simulink model "my_stanley"  (R2020a)
settings: Solver=FixedStepAuto  StartTime=0.0  StopTime=20  FixedStep=.01  RelTol=1e-3
libraries: simulink x2
settings Model: Creator=Jamie  LastModifiedBy=Jamie
settings SolverCC: AlgebraicLoopSolver=LineSearch

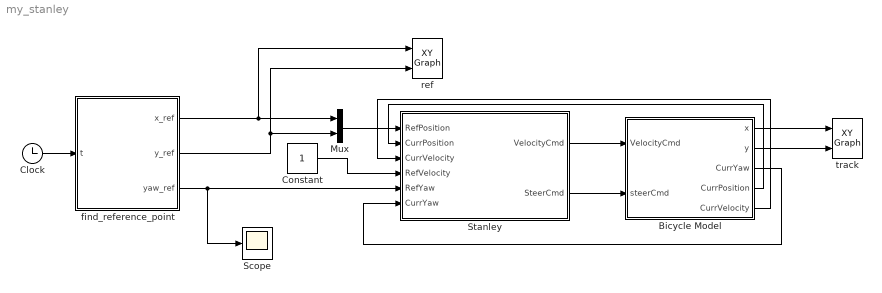
== system my_stanley ==
  Bicycle Model : Subsystem
  Clock : Clock
  Constant : Constant
  Mux : Mux  Inputs=2
  Scope : Scope
  Stanley : Subsystem
  find_reference_point : MATLAB Function  TreatAsAtomicUnit=on
  ref : simulink/Sinks/XY Graph  xmin=-4  xmax=4  ymin=-3  ymax=3  st=-1
  track : simulink/Sinks/XY Graph  xmin=-4  xmax=4  ymin=-3  ymax=3  st=-1
  wires:
  Mux/1 -> Stanley/1(RefPosition)
  Bicycle Model/4(CurrPosition) -> Stanley/2(CurrPosition)
  Stanley/2(SteerCmd) -> Bicycle Model/2(steerCmd)
  Bicycle Model/3(CurrYaw) -> Stanley/6(CurrYaw)
  Bicycle Model/1(x) -> track/1
  Bicycle Model/2(y) -> track/2
  Stanley/1(VelocityCmd) -> Bicycle Model/1(VelocityCmd)
  find_reference_point/1(x_ref) -> ref/1, Mux/1
  find_reference_point/2(y_ref) -> ref/2, Mux/2
  Clock/1 -> find_reference_point/1(t)
  find_reference_point/3(yaw_ref) -> Scope/1, Stanley/5(RefYaw)
  Bicycle Model/5(CurrVelocity) -> Stanley/3(CurrVelocity)
  Constant/1 -> Stanley/4(RefVelocity)

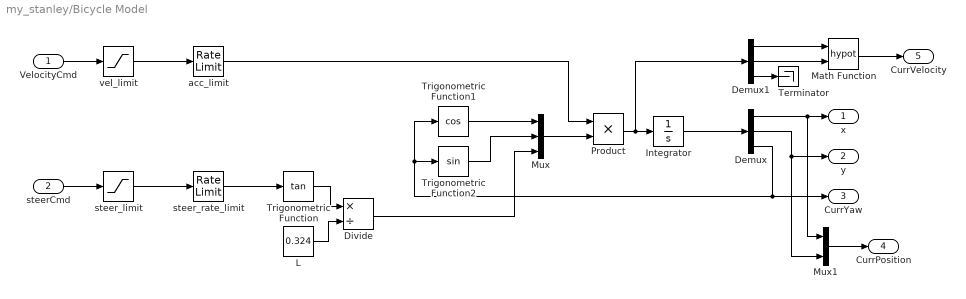
== system my_stanley/Bicycle Model ==
  VelocityCmd : Inport
  steerCmd : Inport  Port=2
  Demux : Demux  Outputs=3
  Demux1 : Demux  Outputs=3
  Divide : Product  Inputs=*/
  Integrator : Integrator  InitialCondition=[0, 0, pi/2]
  L : Constant  Value=0.324
  Math Function : Math  Operator=hypot  SaturateOnIntegerOverflow=on
  Mux : Mux  Inputs=3
  Mux1 : Mux  Inputs=2
  Product : Product
  Terminator : Terminator
  Trigonometric Function : Trigonometry  Operator=tan
  Trigonometric Function1 : Trigonometry  Operator=cos
  Trigonometric Function2 : Trigonometry
  acc_limit : RateLimiter  SampleTimeMode=inherited
  steer_limit : Saturate
  steer_rate_limit : RateLimiter  RisingSlewLimit=3  FallingSlewLimit=-3  SampleTimeMode=inherited
  vel_limit : Saturate  UpperLimit=3  LowerLimit=-3
  x : Outport
  y : Outport  Port=2
  CurrYaw : Outport  Port=3
  CurrPosition : Outport  Port=4
  CurrVelocity : Outport  Port=5
  wires:
  steerCmd/1 -> steer_limit/1
  VelocityCmd/1 -> vel_limit/1
  vel_limit/1 -> acc_limit/1
  steer_limit/1 -> steer_rate_limit/1
  steer_rate_limit/1 -> Trigonometric Function/1
  Trigonometric Function/1 -> Divide/1
  L/1 -> Divide/2
  acc_limit/1 -> Product/1
  Trigonometric Function1/1 -> Mux/1
  Trigonometric Function2/1 -> Mux/2
  Mux/1 -> Product/2
  Product/1 -> Demux1/1, Integrator/1
  Divide/1 -> Mux/3
  Integrator/1 -> Demux/1
  Demux/1 -> Mux1/1, x/1
  Demux/2 -> Mux1/2, y/1
  Demux/3 -> Trigonometric Function1/1, Trigonometric Function2/1, CurrYaw/1
  Mux1/1 -> CurrPosition/1
  Demux1/2 -> Math Function/2
  Demux1/1 -> Math Function/1
  Math Function/1 -> CurrVelocity/1
  Demux1/3 -> Terminator/1

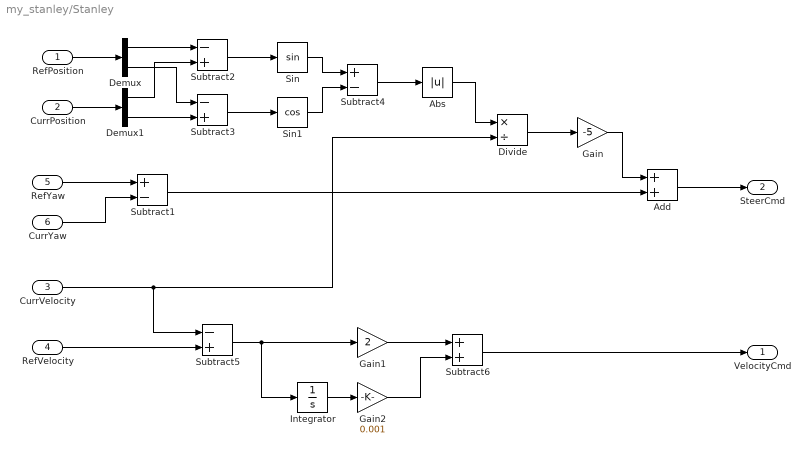
== system my_stanley/Stanley ==
  RefPosition : Inport
  CurrPosition : Inport  Port=2
  CurrVelocity : Inport  Port=3
  RefVelocity : Inport  Port=4
  RefYaw : Inport  Port=5
  CurrYaw : Inport  Port=6
  Abs : Abs
  Add : Sum
  Demux : Demux  Outputs=2
  Demux1 : Demux  Outputs=2
  Divide : Product  Inputs=*/
  Gain : Gain  Gain=-5
  Gain1 : Gain  Gain=2
  Gain2 : Gain  Gain=0.001
  Integrator : Integrator  InitialCondition=0.00001
  Sin : Trigonometry
  Sin1 : Trigonometry  Operator=cos
  Subtract1 : Sum  Inputs=+-
  Subtract2 : Sum  Inputs=-+
  Subtract3 : Sum  Inputs=-+
  Subtract4 : Sum  Inputs=+-
  Subtract5 : Sum  Inputs=-+
  Subtract6 : Sum
  VelocityCmd : Outport
  SteerCmd : Outport  Port=2
  wires:
  RefPosition/1 -> Demux/1
  RefYaw/1 -> Subtract1/1
  CurrYaw/1 -> Subtract1/2
  Add/1 -> SteerCmd/1
  Subtract1/1 -> Add/2
  CurrPosition/1 -> Demux1/1
  Demux1/1 -> Subtract2/2
  Demux/1 -> Subtract2/1
  Subtract2/1 -> Sin/1
  Demux1/2 -> Subtract3/2
  Demux/2 -> Subtract3/1
  Subtract3/1 -> Sin1/1
  Subtract4/1 -> Abs/1
  Sin/1 -> Subtract4/1
  Sin1/1 -> Subtract4/2
  Abs/1 -> Divide/1
  CurrVelocity/1 -> Subtract5/1, Divide/2
  Divide/1 -> Gain/1
  Gain/1 -> Add/1
  RefVelocity/1 -> Subtract5/2
  Subtract5/1 -> Integrator/1, Gain1/1
  Integrator/1 -> Gain2/1
  Subtract6/1 -> VelocityCmd/1
  Gain1/1 -> Subtract6/1
  Gain2/1 -> Subtract6/2

== matlab function my_stanley/find_reference_point ==
  data: t input; x_ref output; y_ref output; yaw_ref output
function [x_ref, y_ref, yaw_ref]= fcn(t)
pi = 3.14159;

v = 1;
R = 1.5;
T0 = pi*R/v;

if (t>4*T0)
    t = mod(t,(4*T0));
end
    
if ((t >= 0)&&(t <= 2*T0))
    x_ref = R + R*cos(pi - (v/R)*t);
    y_ref = R*sin(pi - (v/R)*t);
    yaw_ref = pi/2 - (v/R)*t;
elseif ((t >= 2*T0)&&(t <= 4*T0))
    x_ref = -R - R*cos(pi + (v/R)*(-t + 2*T0));
    y_ref = R*sin(pi + (v/R)*(-t + 2*T0));
    yaw_ref = -3*pi/2 + (v/R)*(t - 2*T0);
else 
    x_ref = 0;
    y_ref = 0;
    yaw_ref = pi/2;
end
